simulink model "MassSpringDamper_ClosedLoop_Reference"  (R2023a)
settings: Solver=ode4  StartTime=0.0  StopTime=5  FixedStep=0.001  RelTol=1e-3
settings Model: Creator=Fasih  LastModifiedBy=Fasih

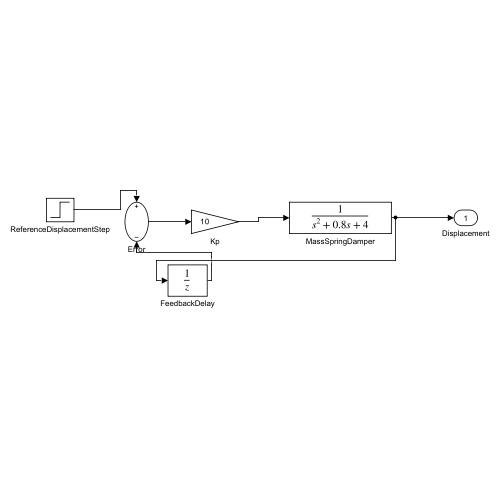
[thumbnail: Simulink's stored preview of the top-level diagram]
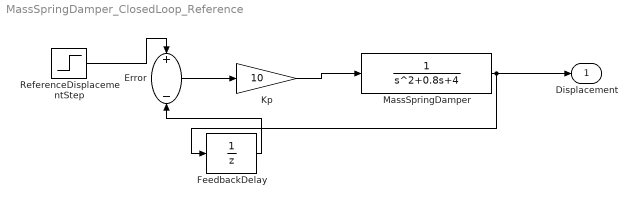
== system MassSpringDamper_ClosedLoop_Reference ==
  Error : Sum  Inputs=+-
  FeedbackDelay : UnitDelay  SampleTime=0.001  HasFrameUpgradeWarning=on
  Kp : Gain  Gain=10
  MassSpringDamper : TransferFcn  Denominator=[1 0.8 4]
  ReferenceDisplacementStep : Step  Time=0  SampleTime=0
  Displacement : Outport
  wires:
  ReferenceDisplacementStep/1 -> Error/1
  FeedbackDelay/1 -> Error/2
  Error/1 -> Kp/1
  Kp/1 -> MassSpringDamper/1
  MassSpringDamper/1 -> Displacement/1, FeedbackDelay/1
